simulink model "MPC3DoF"  (R2025a)
settings: Solver=VariableStepAuto  StartTime=0.0  StopTime=stop_time  RelTol=1e-3
model workspace (MAT data in the model file):
  com_error = 0
  controller_type : ControllerType (value not decoded)
  discrepancy = 0.5
  dtime = 0.3
  enable_turbulence = 0
  g = 9.8
  inertia_error = 0
  mass_error = 0
  max_gimbal_rate = 5
  max_iter = 400
  max_throttle_rate = 0.5
  nominal_val = 5
  optimization_time = 0.3
  steps = 50
  stop_time = 100
  u0 = [0.443891402715 0]
  vehicle = Vehicle
  vehicle.m = 100000
  vehicle.L = 30
  vehicle.I = 30000000
  vehicle.Len = 60
  vehicle.max_gimbal = 0.174532925199
  vehicle.min_thrust = 440000
  vehicle.max_thrust = 2210000
  vehicle.Name = "Astra2"
  x0 = [100 100 0 0 1.57079632679 0]
  xf = [0 0 0 0 1.57079632679 0]
libraries: simulink_extras x4, aerolibanim x1, sharedTrackingLibrary x1, SignalEditorBlockLib x1
settings Model: Creator=alexa  LastModifiedBy=thatf

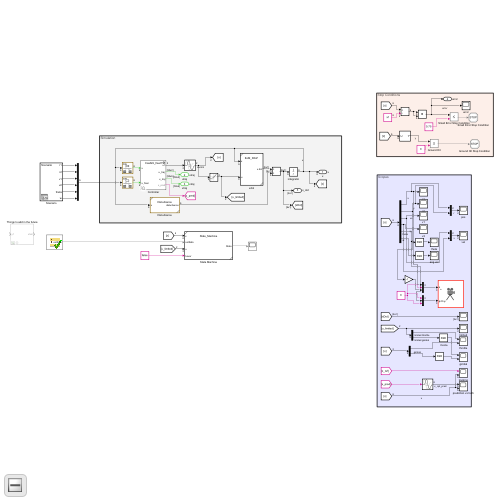
[thumbnail: Simulink's stored preview of the top-level diagram]
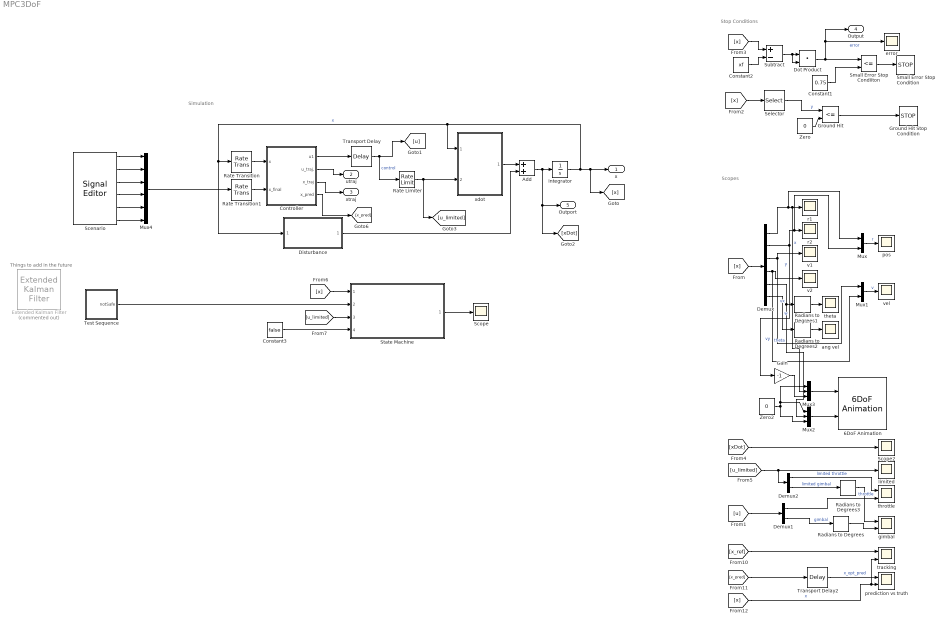
== system MPC3DoF ==
  note: Simulation
  note: Stop Conditions
  note: Things to add in the future
  note: Scopes
  6DoF Animation : aerolibanim/6DoF Animation  u1=[-100 100 -100 100 -800 0]  u2=0.1  u3=10.0  u4=[0, 0, 0]  u5=Fixed position  u6=[0,80,-50]  u7=40  u8=on
  Add : Sum
  Constant1 : Constant  Value=0.75
  Constant2 : Constant  Value=xf
  Constant3 : Constant  Value=false
  Controller : Subsystem  Variant=on  VariantChoicesSpecifier={}  VariantChoicesEnumeration=ControllerType  VariantControlVariable=controller_type
  Demux : Demux  Outputs=6
  Demux1 : Demux  Outputs=2
  Demux2 : Demux  Outputs=2
  Disturbance : Subsystem  ReferencedSubsystem=Disturbance
  Dot Product : DotProduct  OutDataTypeStr=Inherit: Inherit via internal rule
  Extended Kalman Filter : sharedTrackingLibrary/Extended Kalman Filter  Commented=on  StateTransitionFcn=myStateTransitionFcn  HasStateTransitionJacobianFcn=off  HasAdditiveProcessNoise=Additive  ProcessNoise=1  HasTimeVaryingProcessNoise=off  HasStateTransitionFcnExtraArgument=0  InitialState=0  InitialStateCovariance=1  MeasurementFcn1=myMeasurementFcn  HasMeasurementJacobianFcn1=off  HasMeasurementEnablePort1=off  HasAdditiveMeasurementNoise1=Additive  MeasurementNoise1=1  HasTimeVaryingMeasurementNoise1=off  HasMeasurementFcnExtraArgument1=0  HasMeasurementWrapping1=off  MeasurementFcn2=myMeasurementFcn  HasMeasurementJacobianFcn2=off  HasMeasurementEnablePort2=off  HasAdditiveMeasurementNoise2=Additive  MeasurementNoise2=1  HasTimeVaryingMeasurementNoise2=off  HasMeasurementFcnExtraArgument2=0  HasMeasurementWrapping2=off  MeasurementFcn3=myMeasurementFcn  HasMeasurementJacobianFcn3=off  HasMeasurementEnablePort3=off  HasAdditiveMeasurementNoise3=Additive  MeasurementNoise3=1  HasTimeVaryingMeasurementNoise3=off  HasMeasurementFcnExtraArgument3=0  HasMeasurementWrapping3=off  MeasurementFcn4=myMeasurementFcn  HasMeasurementJacobianFcn4=off  HasMeasurementEnablePort4=off  HasAdditiveMeasurementNoise4=Additive  MeasurementNoise4=1  HasTimeVaryingMeasurementNoise4=off  HasMeasurementFcnExtraArgument4=0  HasMeasurementWrapping4=off  MeasurementFcn5=myMeasurementFcn  HasMeasurementJacobianFcn5=off  HasMeasurementEnablePort5=off  HasAdditiveMeasurementNoise5=Additive  MeasurementNoise5=1  HasTimeVaryingMeasurementNoise5=off  HasMeasurementFcnExtraArgument5=0  HasMeasurementWrapping5=off  EnableMultirate=off  StateTransitionFcnSampleTime=1  MeasurementFcn1SampleTime=1  MeasurementFcn2SampleTime=1  MeasurementFcn3SampleTime=1  MeasurementFcn4SampleTime=1  MeasurementFcn5SampleTime=1  UseCurrentEstimator=on  OutputStateCovariance=off  DataType=double  SampleTime=1  NumberOfMeasurements=1
  Gain : Gain  Gain=-1
  Ground Hit : RelationalOperator  Operator=<=  OutDataTypeStr=boolean  RndMeth=Simplest  InputSameDT=off
  Ground Hit Stop Condition : Stop
  Mux : Mux  Inputs=2
  Mux1 : Mux  Inputs=2
  Mux2 : Mux  Inputs=3
  Mux3 : Mux  Inputs=3
  Mux4 : Mux  Inputs=6
  Radians to Degrees{,1..3} (4 alike) : simulink_extras/Transformations/Radians to Degrees
  Rate Limiter : RateLimiter  RisingSlewLimit=[max_throttle_rate max_gimbal_rate]*100  FallingSlewLimit=[-max_throttle_rate -max_gimbal_rate]*100  SampleTimeMode=inherited  InitialCondition=u0
  Rate Transition : RateTransition  InitialCondition=x0  OutPortSampleTime=optimization_time
  Rate Transition1 : RateTransition  InitialCondition=xf  OutPortSampleTime=optimization_time
  Scenario : SignalEditorBlockLib/Signal Editor  FileName=land_at_origin_scenario.mat  ActiveScenario=Scenario  ActiveSignal=w  IsBus=off  OutputBusObjectStr=Bus: BusObject  SampleTime=0  ZeroCross=off  OutputAfterFinalValue=Holding final value  Unit=inherit  PreserveSignalName=on  ApplySigPropsToAllScenarios=on  ApplySigPropsToAllSignals=on  SignalPropertySource=Dialog parameters
  Scope : Scope
      settings: ActiveDisplayYMinimum=0.75  ActiveDisplayYMaximum=3.25  DataLoggingVariableName=ScopeData11
  Scope2 : Scope
      settings: ActiveDisplayYMinimum=-51.1711  ActiveDisplayYMaximum=35.55627  DataLoggingVariableName=ScopeData11
  Selector : Selector  InputPortWidth=6  IndexOptions=Index vector (dialog)  Indices=[2]  OutputSizes=1
  Small Error Stop Condiiton : RelationalOperator  Operator=<=  OutDataTypeStr=boolean  RndMeth=Simplest  InputSameDT=off
  Small Error Stop Condition : Stop
  State Machine : Subsystem  ReferencedSubsystem=State_Machine
  Subtract : Sum  Inputs=+-
  Test Sequence : Test Sequence  TreatAsAtomicUnit=on
  Transport Delay : TransportDelay  DelayTime=optimization_time  InitialOutput=u0
  Transport Delay2 : TransportDelay  DelayTime=optimization_time  InitialOutput=x0'
  Zero : Constant  Value=0  OutDataTypeStr=Inherit: Inherit via back propagation
  Zero2 : Constant  Value=0  OutDataTypeStr=Inherit: Inherit via back propagation
  ang vel : Scope
      settings: ActiveDisplayYMinimum=-2.37191  ActiveDisplayYMaximum=13.59448  DataLoggingVariableName=ScopeData14
  error : Scope
      settings: ActiveDisplayYMinimum=-68.18493  ActiveDisplayYMaximum=209.23133  DataLoggingVariableName=ScopeData2
  gimbal : Scope  NumInputPorts=2
      settings: ActiveDisplayYMinimum=-5.1495195108829144  ActiveDisplayYMaximum=2.5864497007590685  DataLoggingVariableName=ScopeData15
  integrator : Integrator  InitialCondition=x0
  limited : Scope
      settings: ActiveDisplayYMinimum=-0.38121977452963457  ActiveDisplayYMaximum=1.0653194545778477  DataLoggingVariableName=ScopeData16
  pos : Scope
      settings: ActiveDisplayYMinimum=-58.15853  ActiveDisplayYMaximum=450.9065  DataLoggingVariableName=ScopeData17
  prediction vs truth : Scope  NumInputPorts=2
      settings: ActiveDisplayYMinimum=-49.046439679734235  ActiveDisplayYMaximum=121.37045029645144  DataLoggingVariableName=ScopeData18
  r1 : Scope
      settings: ActiveDisplayYMinimum=-3E-15  ActiveDisplayYMaximum=1.4E-14  DataLoggingVariableName=ScopeData19
  r2 : Scope
      settings: ActiveDisplayYMinimum=-1.25  ActiveDisplayYMaximum=11.25  DataLoggingVariableName=ScopeData20
  theta : Scope
      settings: ActiveDisplayYMinimum=52.15485  ActiveDisplayYMaximum=103.56413  DataLoggingVariableName=ScopeData21
  throttle : Scope  NumInputPorts=2
      settings: ActiveDisplayYMinimum=0.09898  ActiveDisplayYMaximum=1.10011  DataLoggingVariableName=ScopeData22
  tracking : Scope  NumInputPorts=2
      settings: ActiveDisplayYMinimum=-36.171702788113379  ActiveDisplayYMaximum=133.92743376513329  DataLoggingVariableName=ScopeData23
  v1 : Scope
      settings: ActiveDisplayYMinimum=-3.8E-15  ActiveDisplayYMaximum=4.2E-15  DataLoggingVariableName=ScopeData24
  v2 : Scope
      settings: ActiveDisplayYMinimum=-2.32296  ActiveDisplayYMaximum=0.25811  DataLoggingVariableName=ScopeData25
  vel : Scope
      settings: ActiveDisplayYMinimum=-1.25712  ActiveDisplayYMaximum=0.7237  DataLoggingVariableName=ScopeData26
  xdot : Subsystem  ReferencedSubsystem=EoM_3DoF
  x : Outport  SignalName=x
  utraj : Outport  Port=2  SignalName=utraj
  xtraj : Outport  Port=3  SignalName=xtraj
  Output : Outport  Port=4  SignalName=error
  Outport : Outport  Port=5  SignalName=x_dot
  wires:
  xdot/1 -> Add/1
  integrator/1 -> Disturbance/1, Rate Transition/1, xdot/1, x/1, [x]  "x"
  Controller/3(x_traj) -> xtraj/1
  Transport Delay/1 -> [u], Rate Limiter/1  "control"
  Controller/2(u_traj.) -> utraj/1
  Add/1 -> integrator/1, [xDot], Outport/1
  Rate Transition/1 -> Controller/1(x)
  Disturbance/1 -> Add/2
  Controller/1(u1) -> Transport Delay/1
  Ground Hit/1 -> Ground Hit Stop Condition/1
  Constant1/1 -> Small Error Stop Condiiton/2
  Constant2/1 -> Subtract/2
  Selector/1 -> Ground Hit/1  "y"
  Dot Product/1 -> Output/1, error/1, Small Error Stop Condiiton/1  "error"
  Subtract/1 -> Dot Product/2, Dot Product/1
  [x] -> Selector/1
  Zero/1 -> Ground Hit/2
  [x] -> Subtract/1
  Small Error Stop Condiiton/1 -> Small Error Stop Condition/1
  Rate Limiter/1 -> [u_limited], xdot/2
  Mux4/1 -> Rate Transition1/1
  Rate Transition1/1 -> Controller/2(x_final)
  Controller/4(x_pred) -> [x_pred]
  Scenario/6 -> Mux4/6
  Scenario/5 -> Mux4/5
  Scenario/4 -> Mux4/4
  Scenario/3 -> Mux4/3
  Scenario/2 -> Mux4/2
  Scenario/1 -> Mux4/1
  Test Sequence/1(notSafe) -> State Machine/2
  [x] -> State Machine/1
  [u_limited] -> State Machine/3
  Constant3/1 -> State Machine/4
  State Machine/1 -> Scope/1
  Zero2/1 -> Mux2/1, Mux3/2, Mux2/3
  Mux2/1 -> 6DoF Animation/2
  [x_ref] -> tracking/1
  Demux/4 -> Mux1/2, v2/1  "vy"
  Radians to Degrees/1 -> gimbal/2
  Mux/1 -> pos/1  "r"
  Demux1/2 -> Radians to Degrees/1  "gimbal"
  Transport Delay2/1 -> prediction vs truth/1  "x_opt_pred"
  Demux/3 -> v1/1, Mux1/1  "vx"
  Demux1/1 -> throttle/2  "throttle"
  [x] -> tracking/2, prediction vs truth/2  "x"
  Gain/1 -> Mux3/3
  Demux/6 -> Radians to Degrees2/1  "w"
  Demux/5 -> Mux2/2, Radians to Degrees1/1  "theta"
  Demux2/2 -> Radians to Degrees3/1  "limited gimbal"
  Demux2/1 -> throttle/1  "limited throttle"
  Mux3/1 -> 6DoF Animation/1
  Radians to Degrees2/1 -> ang vel/1
  Radians to Degrees1/1 -> theta/1
  [x_pred] -> Transport Delay2/1
  Radians to Degrees3/1 -> gimbal/1
  Mux1/1 -> vel/1  "v"
  Demux/1 -> Mux/1, Mux3/1, r1/1  "x"
  [u] -> Demux1/1
  [xDot] -> Scope2/1
  [u_limited] -> Demux2/1, limited/1
  Demux/2 -> Mux/2, r2/1, Gain/1  "y"
  [x] -> Demux/1

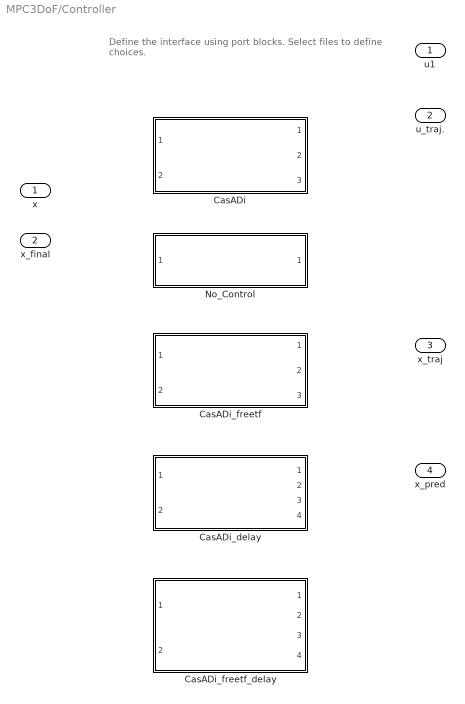
== system MPC3DoF/Controller ==
  note: Define the interface using port blocks.
      | Select files to define choices.
  x : Inport
  x_final : Inport  Port=2
  CasADi : Subsystem  VariantControl=controller_type == ControllerType.CasADi  ReferencedSubsystem=CasADi
  CasADi_delay : Subsystem  VariantControl=controller_type == ControllerType.CasADi_delay  ReferencedSubsystem=CasADi_delay
  CasADi_freetf : Subsystem  VariantControl=controller_type == ControllerType.CasADi_freetf  ReferencedSubsystem=CasADi_freetf
  CasADi_freetf_delay : Subsystem  VariantControl=controller_type == ControllerType.CasADi_freetf_delay  ReferencedSubsystem=CasADi_freetf_delay
  No_Control : Subsystem  VariantControl=controller_type == ControllerType.No_Control  ReferencedSubsystem=No_Control
  u1 : Outport
  u_traj. : Outport  Port=2
  x_traj : Outport  Port=3
  x_pred : Outport  Port=4

== stateflow chart MPC3DoF/Test Sequence ==
  state Scenario_1
    state step_1
    state step_2
      notSafe = true;
    (default) -> step_1
    step_1 -> step_2 : [
        | after(5, sec)
        | ]
  (default) -> Scenario_1 : {assert(Active_Scenario_Index == 1,'The value of Scenario Parameter ''Active_Scenario_Index'' is not valid. Use the index of the scenario to specify it.')}
  data: Active_Scenario_Index parameter =1; notSafe output
